simulink model "compound_pendulum"  (R2018b)
settings: Solver=VariableStepAuto  StartTime=0.0  StopTime=80  RelTol=1e-3
model workspace (MAT data in the model file):
  J = 0.009
  L = 0.495
  c = 0.00035
  d = 0.023
  g = 9.80665
  m = 0.43
libraries: simulink_extras x2, fuzblock x1
settings Model: Creator=jordiae  LastModifiedBy=jordiae
settings SolverCC: ZeroCrossControl=DisableAll
settings OptimizationCC: BooleanDataType=off

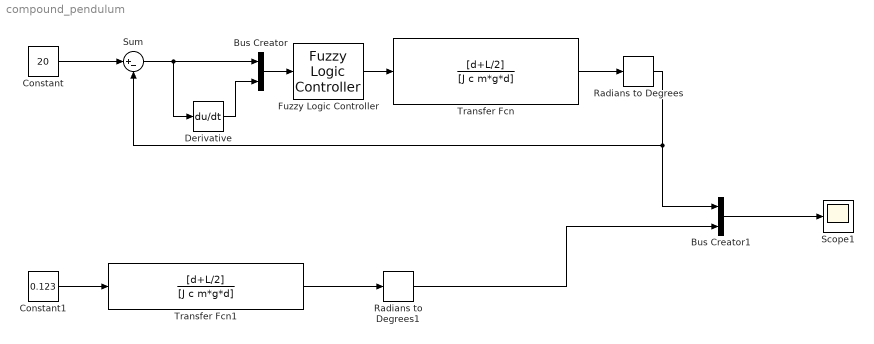
== system compound_pendulum ==
  Bus Creator : BusCreator  Inputs=2
  Bus Creator1 : BusCreator  Inputs=2
  Constant : Constant  Value=20
  Constant1 : Constant  Value=0.123
  Derivative : Derivative
  Fuzzy Logic Controller : fuzblock/Fuzzy Logic  Controller  FIS='pendulum_controller.fis'  OutputSampleNumber=101  DataType=double  FuzzifiedInputs=off  RuleFiringStrengths=off  RuleOutputs=off  AggregatedOutputs=off  SimulateUsing=Interpreted execution  OutOfRangeInputValueMessage=warning  NoRuleFiredMessage=warning  EmptyOutputFuzzySetMessage=warning
  Radians to Degrees : simulink_extras/Transformations/Radians to Degrees
  Radians to Degrees1 : simulink_extras/Transformations/Radians to Degrees
  Scope1 : Scope
  Sum : Sum  Inputs=|+-
  Transfer Fcn : TransferFcn  Numerator=[d+L/2]  Denominator=[J c m*g*d]
  Transfer Fcn1 : TransferFcn  Numerator=[d+L/2]  Denominator=[J c m*g*d]
  wires:
  Constant/1 -> Sum/1
  Sum/1 -> Derivative/1, Bus Creator/1
  Derivative/1 -> Bus Creator/2
  Bus Creator/1 -> Fuzzy Logic Controller/1
  Fuzzy Logic Controller/1 -> Transfer Fcn/1
  Transfer Fcn/1 -> Radians to Degrees/1
  Constant1/1 -> Transfer Fcn1/1
  Transfer Fcn1/1 -> Radians to Degrees1/1
  Bus Creator1/1 -> Scope1/1
  Radians to Degrees/1 -> Bus Creator1/1, Sum/2
  Radians to Degrees1/1 -> Bus Creator1/2
